simulink library "libActions"  (Simulink 8.6)
settings: Solver=VariableStepAuto  StartTime=0.0  StopTime=10.0  RelTol=1e-3
settings Model: Creator=Josef  LastModifiedBy=Josef

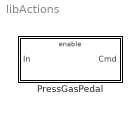
== system libActions ==
  PressGasPedal : Subsystem  TreatAsAtomicUnit=on

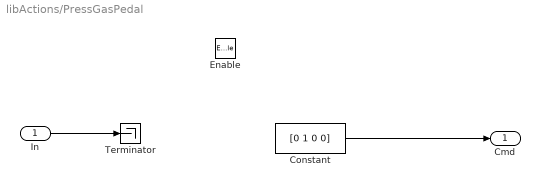
== system libActions/PressGasPedal ==
  In : Inport
  Enable : EnablePort
  Constant : Constant  Value=[0 1 0 0]
  Terminator : Terminator
  Cmd : Outport
  wires:
  In/1 -> Terminator/1
  Constant/1 -> Cmd/1
